simulink model "db"  (R2018a)
settings: Solver=VariableStepAuto  StartTime=0.0  StopTime=60  MaxStep=1e-3  RelTol=1e-3
values from neighbouring files (symbols this model uses):
  h = tf(2,[1 4 8])    [ejemplo_ft.m]
undefined symbols (not defined in the file or in its folder): A, B, C
settings Model: Creator=carma  LastModifiedBy=carma

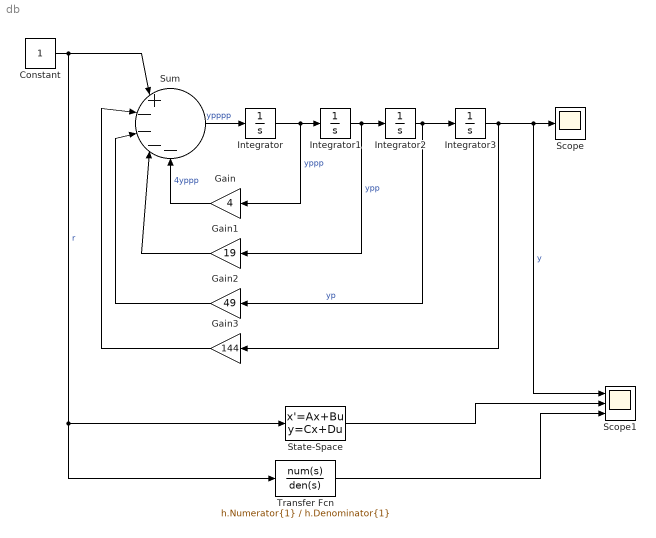
== system db ==
  Constant : Constant
  Gain : Gain  Gain=4
  Gain1 : Gain  Gain=19
  Gain2 : Gain  Gain=49
  Gain3 : Gain  Gain=144
  Integrator{,1..3} (4 alike) : Integrator
  Scope : Scope
  Scope1 : Scope  NumInputPorts=3
  State-Space : StateSpace  A=A  B=B  C=C  D=0  InitialCondition=0
  Sum : Sum  Inputs=|+----
  Transfer Fcn : TransferFcn  Numerator=h.Numerator{1}  Denominator=h.Denominator{1}
  wires:
  Constant/1 -> Transfer Fcn/1, State-Space/1, Sum/1  "r"
  Gain3/1 -> Sum/2
  Gain2/1 -> Sum/3
  Gain1/1 -> Sum/4
  Gain/1 -> Sum/5  "4yppp"
  Sum/1 -> Integrator/1  "ypppp"
  Integrator/1 -> Gain/1, Integrator1/1  "yppp"
  Integrator1/1 -> Gain1/1, Integrator2/1  "ypp"
  Integrator2/1 -> Gain2/1, Integrator3/1  "yp"
  Integrator3/1 -> Gain3/1, Scope1/1, Scope/1  "y"
  State-Space/1 -> Scope1/2
  Transfer Fcn/1 -> Scope1/3
